simulink model "cartpolesystemmodel"  (Simulink 8.7)
settings: Solver=VariableStepAuto  StartTime=0.0  StopTime=10.0  RelTol=1e-3
values from neighbouring files (symbols this model uses):
  g = 9.8    [CartPoleLQR.m]    (also in CartPolePID.m; CartPoleStateSpaceModel.m)
  m = 0.1    [CartPoleLQR.m]    (also in CartPolePID.m; CartPoleStateSpaceModel.m)
  M = 1    [CartPoleLQR.m]    (also in CartPolePID.m; CartPoleStateSpaceModel.m)
undefined symbols (not defined in the file or in its folder): L
settings Model: Creator=spshetty  LastModifiedBy=spshetty
settings DataIOCC: LimitDataPoints=off  SaveFormat=Dataset
settings DebuggingCC: UnderspecifiedInitializationDetection=Simplified  MergeDetectMultiDrivingBlocksExec=error
settings HardwareCC: ProdBitPerPointer=64  ProdLargestAtomicFloat=Float  ProdIntDivRoundTo=Zero  ProdEndianess=LittleEndian  ProdWordSize=64  ProdHWDeviceType=Intel->x86-64 (Windows64)
settings ModelReferenceCC: PropagateSignalLabelsOutOfModel=on
settings ConfigComp: CovModelRefEnable=off

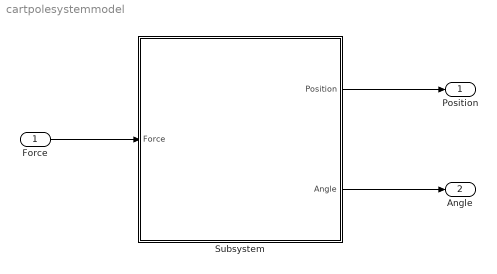
== system cartpolesystemmodel ==
  Force : Inport
  Subsystem : Subsystem
  Position : Outport
  Angle : Outport  Port=2
  wires:
  Force/1 -> Subsystem/1(Force)
  Subsystem/1(Position) -> Position/1
  Subsystem/2(Angle) -> Angle/1

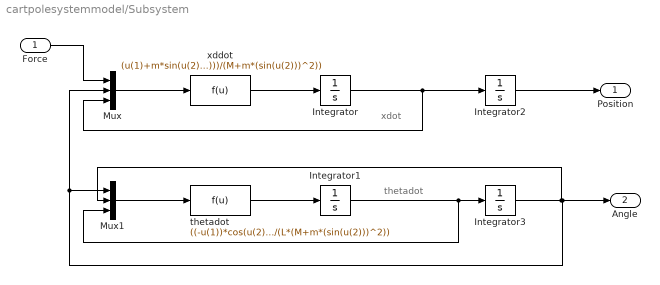
== system cartpolesystemmodel/Subsystem ==
  note: thetadot
  note: xdot
  Force : Inport
  Integrator : Integrator  ContinuousStateAttributes='xdot'
  Integrator1 : Integrator  InitialCondition=pi  ContinuousStateAttributes='thetadot'
  Integrator2 : Integrator  ContinuousStateAttributes='x'
  Integrator3 : Integrator  ContinuousStateAttributes='theta'
  Mux : Mux  Inputs=3
  Mux1 : Mux  Inputs=3
  thetadot : Fcn  Expr=((-u(1))*cos(u(2))-m*L*((u(3))^2)*sin(u(2))*cos(u(2))+(M+m)*g*sin(u(2)))/(L*(M+m*(sin(u(2)))^2))
  xddot : Fcn  Expr=(u(1)+m*sin(u(2))*(L*((u(3))^2)-g*cos(u(2)))/(M+m*(sin(u(2)))^2))
  Position : Outport
  Angle : Outport  Port=2
  wires:
  Mux1/1 -> thetadot/1
  Integrator3/1 -> Angle/1, Mux1/1, Mux/2, Mux1/2
  Mux/1 -> xddot/1
  thetadot/1 -> Integrator1/1
  Integrator1/1 -> Mux1/3, Integrator3/1
  Integrator/1 -> Mux/3, Integrator2/1
  Integrator2/1 -> Position/1
  Force/1 -> Mux/1
  xddot/1 -> Integrator/1
